simulink model "Arrays3_1_tmp"  (Simulink 8.3)
settings: Solver=FixedStepDiscrete  StartTime=0.0  StopTime=10000.0  RelTol=1e-3
settings Model: Creator=scaife  LastModifiedBy=bourbouh  CovSFcnEnable=on  ExtModeAutoUpdateStatusClock=off
settings DataIOCC: SignalLoggingName=sigsOut
settings DebuggingCC: SaveWithParameterizedLinksMsg=none  SignalResolutionControl=TryResolveAllWithWarning  SolverPrmCheckMsg=none  MultiTaskDSMMsg=warning  MultiTaskCondExecSysMsg=none  FrameProcessingCompatibilityMsg=error  StateNameClashWarn=none
settings HardwareCC: TargetUnknown=on
settings SFSimCC: SimParseCustomCode=off
settings GRTTargetCC: GeneratePreprocessorConditionals=Use local settings

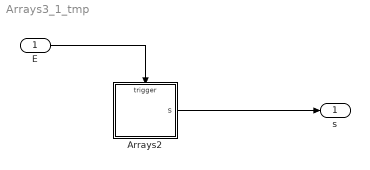
== system Arrays3_1_tmp ==
  E : Inport
  Arrays2 : Stateflow chart  TreatAsAtomicUnit=on
      settings: PermitHierarchicalResolution=ParametersOnly
  s : Outport
  wires:
  E/1 -> Arrays2/Trigger
  Arrays2/1(s) -> s/1

== stateflow chart Arrays2 ==
  state A/
    en:x[1][1][1]++
    x[1][1][2]+=2
    x[1][2][1]+=3
    x[1][2][2]+=4
    s=1
  state B/
    en:x[2][1][1]++
    x[2][1][2]+=2
    x[2][2][1]+=3
    x[2][2][2]+=4
    s = 2
  state C/
    en:x[3][1][1]++
    x[3][1][2]+=2
    x[3][2][1]+=3
    x[3][2][2]+=4
    s = 3
  (default) -> A
  A -> B : E
  C -> A : E
  B -> C : E
  data: x local int32 size=3 2 2 [0..100] =1; s output uint8
  events: E input RISING_EDGE_EVENT
